simulink model "ch7example8"  (Simulink 9.2)
settings: Solver=FixedStepDiscrete  StartTime=0.0  StopTime=100.0  FixedStep=1e-5  RelTol=1e-3  EnableMultiTasking=on
undefined symbols (not defined in the file): rcosine
libraries: dspobslib x1, commrandsrc2 x1, commutil2 x1, dspsigops x1
settings Model: Creator=Administrator  LastModifiedBy=Administrator
settings DataIOCC: SignalLoggingName=sigsOut
settings OptimizationCC: LifeSpan=auto
settings DebuggingCC: SaveWithParameterizedLinksMsg=none  SignalResolutionControl=TryResolveAllWithWarning  MultiTaskDSMMsg=warning  MultiTaskCondExecSysMsg=none  FcnCallInpInsideContextMsg=error  StateNameClashWarn=none  SFUnexpectedBacktrackingDiag=error  SFNoUnconditionalDefaultTransitionDiag=error  SFExecutionAtInitializationDiag=warning
settings HardwareCC: TargetUnknown=on
settings SFSimCC: SimUseLocalCustomCode=on
settings RTWCC: RTWUseLocalCustomCode=on
settings CodeAppCC: StateflowObjectComments=off
settings GRTTargetCC: TargetLangStandard=C99 (ISO)  GeneratePreprocessorConditionals=Use local settings
settings ConfigComp: CovExternalEMLEnable=on

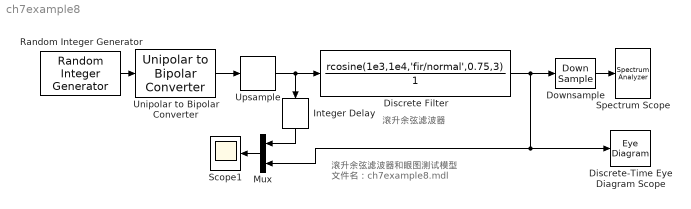
== system ch7example8 ==
  note: 滚升余弦滤波器和眼图测试模型
      | 文件名：ch7example8.mdl
  note: 滚升余弦滤波器
  Discrete Filter : DiscreteFilter  Numerator=rcosine(1e3,1e4,'fir/normal',0.75,3)  Denominator=1
  Discrete-Time Eye Diagram Scope : EyeDiagram  Tag=EyeDiagram
  Downsample : DownSample  N=4  InputProcessing=Inherited (this choice will be removed - see release notes)  RateOptions=Allow multirate processing
  Integer Delay : dspobslib/Integer Delay  delay=30  ic=0  reset_popup=None
      settings: SourceProductName=DSP System Toolbox  SourceProductBaseCode=DS
  Mux : Mux  Inputs=2
  Random Integer Generator : commrandsrc2/Random Integer Generator  mul=4  seed=37  Ts=1e-3  frameBased=off  sampPerFrame=1  orient=off  outDataType=double
  Scope1 : Scope
  Spectrum Scope : SpectrumAnalyzer
  Unipolar to Bipolar Converter : commutil2/Unipolar to Bipolar Converter  M=4  polarity=Positive  dataType=Inherit via internal rule
      settings: SourceProductName=Communications Toolbox
  Upsample : dspsigops/Upsample  N=10  phase=0  InputProcessing=Columns as channels (frame based)  RateOptions=Allow multirate processing  ic=0  mode=Unused parameter value
  wires:
  Unipolar to Bipolar Converter/1 -> Upsample/1
  Upsample/1 -> Discrete Filter/1, Integer Delay/1
  Downsample/1 -> Spectrum Scope/1
  Mux/1 -> Scope1/1
  Integer Delay/1 -> Mux/1
  Random Integer Generator/1 -> Unipolar to Bipolar Converter/1
  Discrete Filter/1 -> Downsample/1, Discrete-Time Eye Diagram Scope/1, Mux/2
